simulink model "deedemo3"  (Simulink 3.00)
settings: Solver=ode45  SolverMode=SingleTasking  StartTime=0.0  StopTime=99999999999  RelTol=1e-3  AbsTol=1e-6
PreLoadFcn:
  | masspgi
undefined symbols (not defined in the file or in its folder): a, k, m
settings Model: SaveTime=off  SaveOutput=off  Creator=sanjai  LastModifiedBy=sanjai

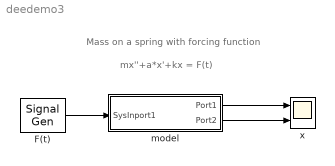
== system deedemo3 ==
  note: mx''+a*x'+kx = F(t)
  note: Mass on a spring with forcing function
  F(t) : SignalGenerator  WaveForm=square  Amplitude=1.000000  Frequency=0.010000  Units=rad/sec
  model : Subsystem
      settings: OpenFcn=diffeqed
      mask Type: Differential Equation Editor (DEE)
      mask Display: disp('mass_on_a_spring')
  x : Scope  NumInputPorts=2
      settings: TickLabels=on  TimeRange=100  YMin=-18~-5  YMax=18~5  SaveToWorkspace=off  SaveName=ScopeData  DataFormat=Matrix
  wires:
  F(t)/1 -> model/1(SysInport1)
  model/1(Port1) -> x/1
  model/2(Port2) -> x/2

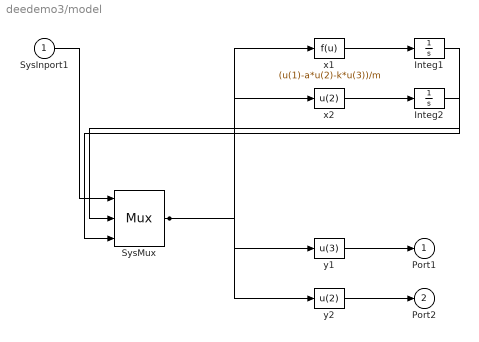
== system deedemo3/model ==
  SysInport1 : Inport  Port=1  PortWidth=-1  SampleTime=-1  DataType=auto
      settings: SignalType=auto
  Integ1 : Integrator  ExternalReset=none  InitialConditionSource=internal  InitialCondition=-1  LimitOutput=off  UpperSaturationLimit=inf  LowerSaturationLimit=-inf  ShowSaturationPort=off  ShowStatePort=off  AbsoluteTolerance=auto
  Integ2 : Integrator  ExternalReset=none  InitialConditionSource=internal  InitialCondition=0  LimitOutput=off  UpperSaturationLimit=inf  LowerSaturationLimit=-inf  ShowSaturationPort=off  ShowStatePort=off  AbsoluteTolerance=auto
  SysMux : Mux  Inputs=3
      settings: DisplayOption=none
  x1 : Fcn  Expr=(u(1)-a*u(2)-k*u(3))/m
  x2 : Fcn  Expr=u(2)
  y1 : Fcn  Expr=u(3)
  y2 : Fcn  Expr=u(2)
  Port1 : Outport  Port=1  InitialOutput=0
  Port2 : Outport  Port=2  InitialOutput=0
  wires:
  y2/1 -> Port2/1
  SysMux/1 -> y2/1, y1/1, x2/1, x1/1
  y1/1 -> Port1/1
  Integ2/1 -> SysMux/3
  x2/1 -> Integ2/1
  Integ1/1 -> SysMux/2
  x1/1 -> Integ1/1
  SysInport1/1 -> SysMux/1
